simulink model "Messages1_2018a"  (R2020b)
settings: Solver=VariableStepAuto  StartTime=0.0  StopTime=0.3  RelTol=1e-3
settings Model: Creator=86188  LastModifiedBy=apple
settings DataIOCC: ReturnWorkspaceOutputs=off
settings DebuggingCC: ArithmeticOperatorsInVariantConditions=warning
settings SFSimCC: SimUseLocalCustomCode=off  CustomCodeUndefinedFunction=UseInterfaceOnly
settings RTWCC: RTWUseLocalCustomCode=off

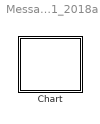
== system Messages1_2018a ==
  Chart : Stateflow chart  TreatAsAtomicUnit=on

== stateflow chart Messages1_2018a/Chart ==
  state A
    en:M.data=3;
    send(M);
  state C
  state D
  state B
  (default) -> A
  C -> D : M
  B -> C : [M.data>0]
  A -> B : M[M.data==3]
  data: M local
